simulink model "MultipleBangBang"  (R2017b)
settings: Solver=VariableStepAuto  StartTime=0.0  StopTime=100.0  RelTol=1e-3
settings Model: Creator=barbot  LastModifiedBy=barbot

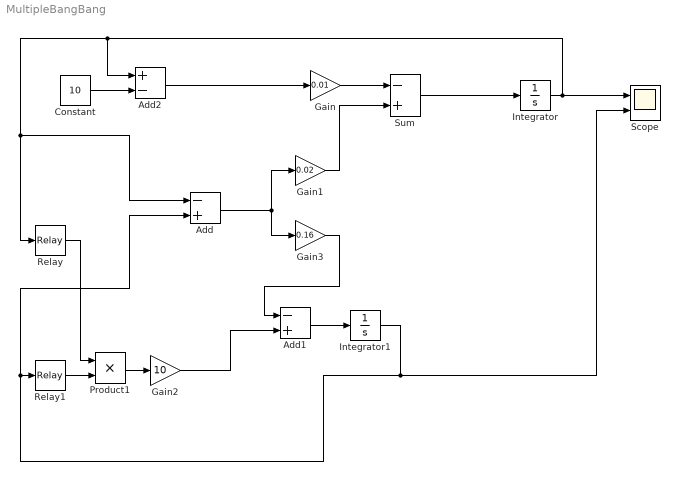
== system MultipleBangBang ==
  Add : Sum  Inputs=-+
  Add1 : Sum  Inputs=-+
  Add2 : Sum  Inputs=+-
  Constant : Constant  Value=10
  Gain : Gain  Gain=0.01
  Gain1 : Gain  Gain=0.02
  Gain2 : Gain  Gain=10
  Gain3 : Gain  Gain=0.16
  Integrator : Integrator  InitialCondition=20
  Integrator1 : Integrator  InitialCondition=20
  Product1 : Product
  Relay : Relay  OnSwitchValue=21  OffSwitchValue=19  OnOutputValue=0  OffOutputValue=1
  Relay1 : Relay  OnSwitchValue=35  OffSwitchValue=30  OnOutputValue=0  OffOutputValue=1
  Scope : Scope  NumInputPorts=2
  Sum : Sum  Inputs=-+
  wires:
  Sum/1 -> Integrator/1
  Integrator/1 -> Add/1, Relay/1, Add2/1, Scope/1
  Gain/1 -> Sum/1
  Relay/1 -> Product1/1
  Gain1/1 -> Sum/2
  Add/1 -> Gain1/1, Gain3/1
  Integrator1/1 -> Add/2, Relay1/1, Scope/2
  Relay1/1 -> Product1/2
  Gain2/1 -> Add1/2
  Add1/1 -> Integrator1/1
  Product1/1 -> Gain2/1
  Gain3/1 -> Add1/1
  Constant/1 -> Add2/2
  Add2/1 -> Gain/1
